simulink model "pid_simu"  (R2021a)
settings: Solver=ode4  StartTime=0.0  StopTime=10  FixedStep=1e-3  RelTol=1e-3
model workspace (MAT data in the model file):
  init_t = 1
libraries: cstblocks x2, simulink x1
settings Model: Creator=rocio  LastModifiedBy=rocio

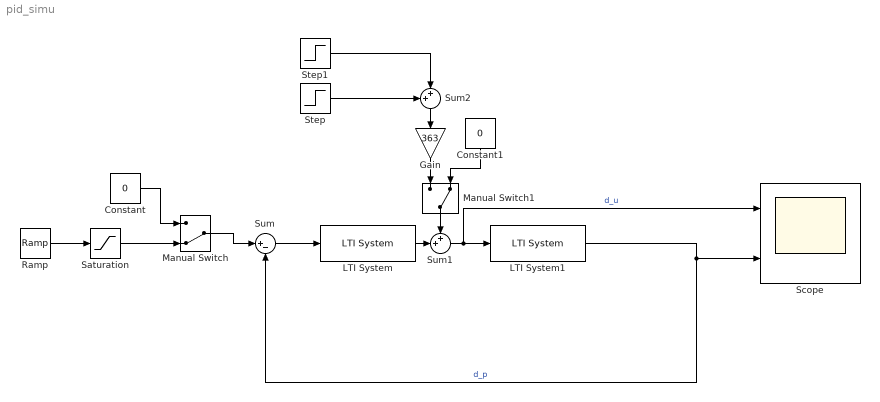
== system pid_simu ==
  Constant : Constant  Value=0
  Constant1 : Constant  Value=0
  Gain : Gain  Gain=363
  LTI System : cstblocks/LTI System  sys=Cd  IC=[]
  LTI System1 : cstblocks/LTI System  sys=P  IC=[]
  Manual Switch : ManualSwitch  CurrentSetting=0
  Manual Switch1 : ManualSwitch  CurrentSetting=0
  Ramp : simulink/Sources/Ramp  slope=10/0.4  start=0  InitialOutput=0
  Saturation : Saturate  UpperLimit=10  LowerLimit=0
  Scope : Scope  NumInputPorts=2
  Step : Step  SampleTime=0
  Step1 : Step  Time=1.4  After=-1  SampleTime=0
  Sum : Sum  Inputs=|+-
  Sum1 : Sum  Inputs=++|
  Sum2 : Sum  Inputs=++|
  wires:
  Sum/1 -> LTI System/1
  LTI System1/1 -> Sum/2, Scope/2  "d_p"
  LTI System/1 -> Sum1/2
  Sum1/1 -> Scope/1, LTI System1/1  "d_u"
  Step/1 -> Sum2/1
  Step1/1 -> Sum2/2
  Manual Switch/1 -> Sum/1
  Constant/1 -> Manual Switch/1
  Manual Switch1/1 -> Sum1/1
  Constant1/1 -> Manual Switch1/2
  Sum2/1 -> Gain/1
  Gain/1 -> Manual Switch1/1
  Ramp/1 -> Saturation/1
  Saturation/1 -> Manual Switch/2
